simulink model "Local_trajectory_export"  (R2021a)
settings: configuration reference "AION_IDS_Speedgoat" (kept outside this file)
undefined symbols (not defined in the file): LATERAL_DISTANCE_THRESHOLD, MAX_GLOBAL_TRAJECTORY_WAY_POINT_NUMBER, MAX_LOCAL_TRAJECTORY_WAY_POINT_NUMBER, MAX_TRAJECTORY_LENGTH, START_END_DISTANCE_THRESHOLD
libraries: simulink x1
(part 1 of 2)
Description:
  | 局部轨迹导出模型
settings Model: DataDictionary=Local_Trajectory_Export.sldd  Creator=xinrui  LastModifiedBy=Administrator
settings ConfigSetRef: SourceName=AION_IDS_Speedgoat

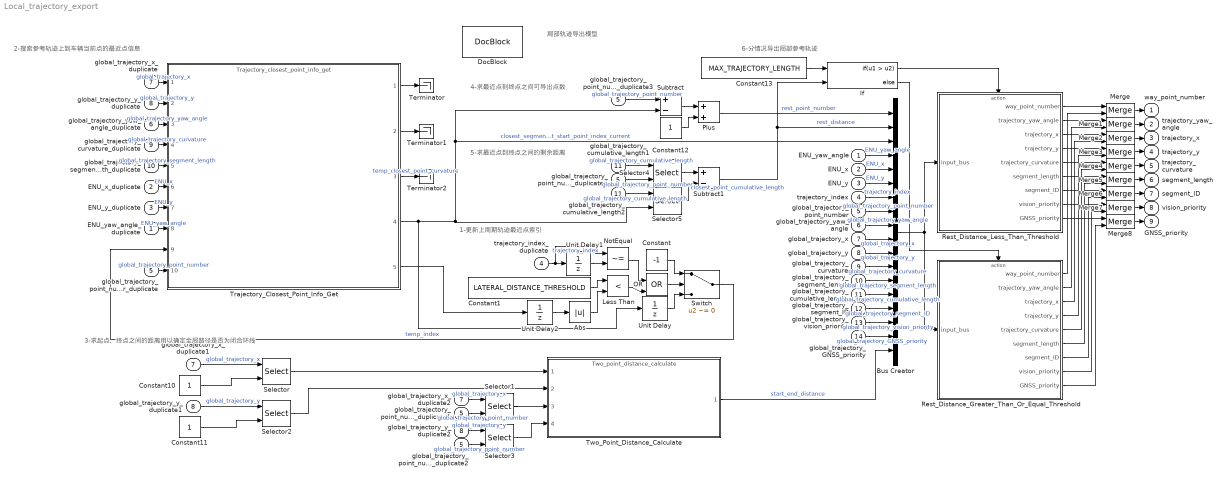
== system Local_trajectory_export ==
  note: 6-分情况导出局部参考轨迹
  note: 5-求最近点到终点之间的剩余距离
  note: 4-求最近点到终点之间可导出点数
  note: 1-更新上周期轨迹最近点索引
  note: 3-求起点、终点之间的距离用以确定全局路径是否为闭合环线
  note: 2-搜索参考轨迹上到车辆当前点的最近点信息
  note: 局部轨迹导出模型
  ENU_yaw_angle : Inport  Description=东北天坐标系下当前点横摆角，实数，deg。  OutDataTypeStr=double  PortDimensions=1
  ENU_x : Inport  Description=东北天坐标系下当前点x坐标，实数，m。  Port=2  OutDataTypeStr=double  PortDimensions=1
  ENU_y : Inport  Description=东北天坐标系下当前点y坐标，实数，m。  Port=3  OutDataTypeStr=double  PortDimensions=1
  trajectory_index : Inport  Description=选择的参考轨迹索引，正整数，无量纲。  Port=4  OutDataTypeStr=int8  PortDimensions=1
  global_trajectory_point_number : Inport  Description=选择的全局参考轨迹路点数量，正整数，无量纲。  Port=5  OutDataTypeStr=int32  PortDimensions=1
  global_trajectory_yaw_angle : Inport  Description=选择的全局参考轨迹横摆角数组，有效数据量为global_trajectory_point_number，实数，deg。  Port=6  OutDataTypeStr=double  PortDimensions=MAX_GLOBAL_TRAJECTORY_WAY_POINT_NUMBER  Interpolate=off
  global_trajectory_x : Inport  Description=选择的全局参考轨迹x坐标数组，有效数据量为global_trajectory_point_number，实数，m。  Port=7  OutDataTypeStr=double  PortDimensions=MAX_GLOBAL_TRAJECTORY_WAY_POINT_NUMBER  Interpolate=off
  global_trajectory_y : Inport  Description=选择的全局参考轨迹y坐标数组，有效数据量为global_trajectory_point_number，实数，m。  Port=8  OutDataTypeStr=double  PortDimensions=MAX_GLOBAL_TRAJECTORY_WAY_POINT_NUMBER  Interpolate=off
  global_trajectory_curvature : Inport  Description=选择的全局参考轨迹曲率数组，有效数据量为global_trajectory_point_number，实数，1/m。  Port=9  OutDataTypeStr=double  PortDimensions=MAX_GLOBAL_TRAJECTORY_WAY_POINT_NUMBER  Interpolate=off
  global_trajectory_segment_length : Inport  Description=选择的全局参考轨迹路点到前一个点的线段长度数组，有效数据量为global_trajectory_point_number，正实数，m。  Port=10  OutDataTypeStr=double  PortDimensions=MAX_GLOBAL_TRAJECTORY_WAY_POINT_NUMBER  Interpolate=off
  global_trajectory_cumulative_length : Inport  Description=选择的全局参考轨迹路点到起点的累计长度数组，有效数据量为global_trajectory_point_number，正实数，m。  Port=11  OutDataTypeStr=double  PortDimensions=MAX_GLOBAL_TRAJECTORY_WAY_POINT_NUMBER  Interpolate=off
  global_trajectory_segment_ID : Inport  Description=选择的全局参考轨迹区间代号数组，有效数据量为global_trajectory_point_number，正整数，无量纲。  Port=12  OutDataTypeStr=int8  PortDimensions=MAX_GLOBAL_TRAJECTORY_WAY_POINT_NUMBER  Interpolate=off
  global_trajectory_vision_priority : Inport  Description=选择的全局参考轨迹视觉循迹优先级数组，有效数据量为global_trajectory_point_number，自然数，无量纲。  Port=13  OutDataTypeStr=int8  PortDimensions=MAX_GLOBAL_TRAJECTORY_WAY_POINT_NUMBER  Interpolate=off
  global_trajectory_GNSS_priority : Inport  Description=选择的全局参考轨迹GNSS循迹优先级数组，有效数据量为global_trajectory_point_number，自然数，无量纲。  Port=14  OutDataTypeStr=int8  PortDimensions=MAX_GLOBAL_TRAJECTORY_WAY_POINT_NUMBER  Interpolate=off
  Abs : Abs
  Bus Creator : BusCreator  Inputs=18
  Constant : Constant  Value=-1  OutDataTypeStr=int32  SampleTime=-1
  Constant1 : Constant  Value=LATERAL_DISTANCE_THRESHOLD  OutDataTypeStr=double  SampleTime=-1
  Constant10 : Constant  OutDataTypeStr=int32  SampleTime=-1
  Constant11 : Constant  OutDataTypeStr=int32  SampleTime=-1
  Constant12 : Constant  OutDataTypeStr=int32  SampleTime=-1
  Constant13 : Constant  Value=MAX_TRAJECTORY_LENGTH  OutDataTypeStr=double  SampleTime=-1
  DocBlock : simulink/Model-Wide Utilities/DocBlock  DocumentType=HTML  mask(DocBlock){}
      mask Display:
      | plot([.8 0 0 1 1 .8 .8 1],[1 1 0 0 .8 1 .8 .8]);
      | text(.5,.6,'CHANGELOG','horizontalalignment','center');
      | text(.95,.05,get_param(gcb,'DocumentType'),'verticalalignment','bottom','horizontalalignment','right');
  ENU_x_duplicate : InportShadow  Description=东北天坐标系下当前点x坐标，实数，m。  Port=2  OutDataTypeStr=double  PortDimensions=1
  ENU_y_duplicate : InportShadow  Description=东北天坐标系下当前点y坐标，实数，m。  Port=3  OutDataTypeStr=double  PortDimensions=1
  ENU_yaw_angle_duplicate : InportShadow  Description=东北天坐标系下当前点横摆角，实数，deg。  OutDataTypeStr=double  PortDimensions=1
  If : If  Description=当最近点到终点之间累计距离不足最大轨迹长度的时候，判断起点、终点之间的距离。  NumInputs=2  IfExpression=u1 > u2
  Less Than : RelationalOperator  Operator=<  OutDataTypeStr=boolean  RndMeth=Simplest
  Merge{,1..8} (9 alike) : Merge
  NotEqual : RelationalOperator  Operator=~=  OutDataTypeStr=boolean  RndMeth=Simplest
  OR : Logic  Operator=OR  IconShape=distinctive  AllPortsSameDT=off  OutDataTypeStr=boolean
  Plus : Sum  Description=求最近点到终点之间可导出点数。
  Rest_Distance_Greater_Than_Or_Equal_Threshold : Subsystem  Description=当最近点到终点之间的累计距离大于最大轨迹长度的时候，按最大轨迹长度导出轨迹。  TreatAsAtomicUnit=on
  Rest_Distance_Less_Than_Threshold : Subsystem  Description=当最近点到终点之间累计距离不足最大轨迹长度的时候，判断起点、终点之间的距离。  TreatAsAtomicUnit=on
  Selector : Selector  Description=获取参考轨迹起点x坐标。  IndexOptions=Index vector (port)  Indices=[1 3]  OutputSizes=1
  Selector1 : Selector  Description=获取参考轨迹终点x坐标。  IndexOptions=Index vector (port)  Indices=[1 3]  OutputSizes=1
  Selector2 : Selector  Description=获取参考轨迹起点y坐标。  IndexOptions=Index vector (port)  Indices=[1 3]  OutputSizes=1
  Selector3 : Selector  Description=获取参考轨迹终点y坐标。  IndexOptions=Index vector (port)  Indices=[1 3]  OutputSizes=1
  Selector4 : Selector  Description=获取参考轨迹终点处的累计长度。  IndexOptions=Index vector (port)  Indices=[1 3]  OutputSizes=1
  Selector5 : Selector  Description=获取参考轨迹最近线段起始点处的累计长度。  IndexOptions=Index vector (port)  Indices=[1 3]  OutputSizes=1
  Subtract : Sum  Inputs=+-
  Subtract1 : Sum  Description=求最近点到终点之间的剩余距离。  Inputs=+-
  Switch : Switch  Description=|  Criteria=u2 ~= 0
      | 当以下任意条件满足时，采用全局搜索最近点，输入索引设置为-1，否则采用上周期的最近线段起始点索引作为本周期输入索引，使用局部搜索最近点信息。
      | （1）选定参考轨迹索引发生改变。
      | （2）近处横向偏差的绝对值大于阈值。
  Terminator : Terminator
  Terminator1 : Terminator
  Terminator2 : Terminator
  Trajectory_Closest_Point_Info_Get : ModelReference  Description=获取所选参考轨迹上的最近点信息。  ModelNameDialog=Trajectory_closest_point_info_get  SimulationMode=Normal  ModelReferenceVersion=4.338
  Two_Point_Distance_Calculate : ModelReference  Description=计算所选参考轨迹的起点和终点之间的距离，以判断参考轨迹是否为闭合环线。  ModelNameDialog=Two_point_distance_calculate  SimulationMode=Normal  ModelReferenceVersion=4.61
  Unit Delay : UnitDelay  InitialCondition=-1  SampleTime=-1  StateName=closest_segment_start_point_index_previous  HasFrameUpgradeWarning=on  StateMustResolveToSignalObject=on
  Unit Delay1 : UnitDelay  InitialCondition=-1  SampleTime=-1  StateName=trajectory_index_previous  HasFrameUpgradeWarning=on  StateMustResolveToSignalObject=on
  Unit Delay2 : UnitDelay  SampleTime=-1  StateName=near_lateral_offset_previous  HasFrameUpgradeWarning=on  StateMustResolveToSignalObject=on
  global_trajectory_cumulative_length1 : InportShadow  Description=选择的全局参考轨迹路点到起点的累计长度数组，有效数据量为global_trajectory_point_number，正实数，m。  Port=11  OutDataTypeStr=double  PortDimensions=MAX_GLOBAL_TRAJECTORY_WAY_POINT_NUMBER  Interpolate=off
  global_trajectory_cumulative_length2 : InportShadow  Description=选择的全局参考轨迹路点到起点的累计长度数组，有效数据量为global_trajectory_point_number，正实数，m。  Port=11  OutDataTypeStr=double  PortDimensions=MAX_GLOBAL_TRAJECTORY_WAY_POINT_NUMBER  Interpolate=off
  global_trajectory_curvature_duplicate : InportShadow  Description=选择的全局参考轨迹曲率数组，有效数据量为global_trajectory_point_number，实数，1/m。  Port=9  OutDataTypeStr=double  PortDimensions=MAX_GLOBAL_TRAJECTORY_WAY_POINT_NUMBER  Interpolate=off
  global_trajectory_point_number_duplicate{,1..4} (5 alike) : InportShadow  Description=选择的全局参考轨迹路点数量，正整数，无量纲。  Port=5  OutDataTypeStr=int32  PortDimensions=1
  global_trajectory_segment_length_duplicate : InportShadow  Description=选择的全局参考轨迹路点到前一个点的线段长度数组，有效数据量为global_trajectory_point_number，正实数，m。  Port=10  OutDataTypeStr=double  PortDimensions=MAX_GLOBAL_TRAJECTORY_WAY_POINT_NUMBER  Interpolate=off
  global_trajectory_x_duplicate : InportShadow  Description=选择的全局参考轨迹x坐标数组，有效数据量为global_trajectory_point_number，实数，m。  Port=7  OutDataTypeStr=double  PortDimensions=MAX_GLOBAL_TRAJECTORY_WAY_POINT_NUMBER  Interpolate=off
  global_trajectory_x_duplicate1 : InportShadow  Description=选择的全局参考轨迹x坐标数组，有效数据量为global_trajectory_point_number，实数，m。  Port=7  OutDataTypeStr=double  PortDimensions=MAX_GLOBAL_TRAJECTORY_WAY_POINT_NUMBER  Interpolate=off
  global_trajectory_x_duplicate2 : InportShadow  Description=选择的全局参考轨迹x坐标数组，有效数据量为global_trajectory_point_number，实数，m。  Port=7  OutDataTypeStr=double  PortDimensions=MAX_GLOBAL_TRAJECTORY_WAY_POINT_NUMBER  Interpolate=off
  global_trajectory_y_duplicate : InportShadow  Description=选择的全局参考轨迹y坐标数组，有效数据量为global_trajectory_point_number，实数，m。  Port=8  OutDataTypeStr=double  PortDimensions=MAX_GLOBAL_TRAJECTORY_WAY_POINT_NUMBER  Interpolate=off
  global_trajectory_y_duplicate1 : InportShadow  Description=选择的全局参考轨迹y坐标数组，有效数据量为global_trajectory_point_number，实数，m。  Port=8  OutDataTypeStr=double  PortDimensions=MAX_GLOBAL_TRAJECTORY_WAY_POINT_NUMBER  Interpolate=off
  global_trajectory_y_duplicate2 : InportShadow  Description=选择的全局参考轨迹y坐标数组，有效数据量为global_trajectory_point_number，实数，m。  Port=8  OutDataTypeStr=double  PortDimensions=MAX_GLOBAL_TRAJECTORY_WAY_POINT_NUMBER  Interpolate=off
  global_trajectory_yaw_angle_duplicate : InportShadow  Description=选择的全局参考轨迹横摆角数组，有效数据量为global_trajectory_point_number，实数，deg。  Port=6  OutDataTypeStr=double  PortDimensions=MAX_GLOBAL_TRAJECTORY_WAY_POINT_NUMBER  Interpolate=off
  trajectory_index_duplicate : InportShadow  Description=选择的参考轨迹索引，正整数，无量纲。  Port=4  OutDataTypeStr=int8  PortDimensions=1
  way_point_number : Outport  Description=导出的局部轨迹有效路点个数，自然数，无量纲。  OutDataTypeStr=int32  PortDimensions=1
  trajectory_yaw_angle : Outport  Description=导出的局部轨迹横摆角数组，有效数据数量为way_point_number，其余补零，实数，deg。  Port=2  OutDataTypeStr=double  PortDimensions=MAX_LOCAL_TRAJECTORY_WAY_POINT_NUMBER
  trajectory_x : Outport  Description=导出的局部轨迹x坐标数组，有效数据数量为way_point_number，其余补零，实数，m。  Port=3  OutDataTypeStr=double  PortDimensions=MAX_LOCAL_TRAJECTORY_WAY_POINT_NUMBER
  trajectory_y : Outport  Description=导出的局部轨迹y坐标数组，有效数据数量为way_point_number，其余补零，实数，m。  Port=4  OutDataTypeStr=double  PortDimensions=MAX_LOCAL_TRAJECTORY_WAY_POINT_NUMBER
  trajectory_curvature : Outport  Description=导出的局部轨迹曲率数组，有效数据数量为way_point_number，其余补零，实数，1/m。  Port=5  OutDataTypeStr=double  PortDimensions=MAX_LOCAL_TRAJECTORY_WAY_POINT_NUMBER
  segment_length : Outport  Description=导出的局部轨迹路点到前一个点的线段长度数组，有效数据数量为way_point_number，其余补零，正实数，m。  Port=6  OutDataTypeStr=double  PortDimensions=MAX_LOCAL_TRAJECTORY_WAY_POINT_NUMBER
  segment_ID : Outport  Description=导出的局部轨迹区间代号数组，有效数据数量为way_point_number，其余补零，正整数，无量纲。  Port=7  OutDataTypeStr=int8  PortDimensions=MAX_LOCAL_TRAJECTORY_WAY_POINT_NUMBER
  vision_priority : Outport  Description=导出的局部轨迹视觉循迹优先级数组，有效数据数量为way_point_number，其余补零，自然数，无量纲。  Port=8  OutDataTypeStr=int8  PortDimensions=MAX_LOCAL_TRAJECTORY_WAY_POINT_NUMBER
  GNSS_priority : Outport  Description=导出的局部轨迹GNSS循迹优先级数组，有效数据数量为way_point_number，其余补零，自然数，无量纲。  Port=9  OutDataTypeStr=int8  PortDimensions=MAX_LOCAL_TRAJECTORY_WAY_POINT_NUMBER
  wires:
  trajectory_index_duplicate/1 -> NotEqual/1, Unit Delay1/1  "trajectory_index"
  Switch/1 -> Trajectory_Closest_Point_Info_Get/9  "temp_index"
  Constant/1 -> Switch/1
  Trajectory_Closest_Point_Info_Get/4 -> Unit Delay/1, Subtract/2, Bus Creator/3, Selector5/2  "closest_segment_start_point_index_current"
  Unit Delay/1 -> Switch/3
  global_trajectory_x_duplicate/1 -> Trajectory_Closest_Point_Info_Get/1  "global_trajectory_x"
  global_trajectory_y_duplicate/1 -> Trajectory_Closest_Point_Info_Get/2  "global_trajectory_y"
  global_trajectory_yaw_angle_duplicate/1 -> Trajectory_Closest_Point_Info_Get/3  "global_trajectory_yaw_angle"
  global_trajectory_curvature_duplicate/1 -> Trajectory_Closest_Point_Info_Get/4  "global_trajectory_curvature"
  global_trajectory_segment_length_duplicate/1 -> Trajectory_Closest_Point_Info_Get/5  "global_trajectory_segment_length"
  ENU_x_duplicate/1 -> Trajectory_Closest_Point_Info_Get/6  "ENU_x"
  ENU_y_duplicate/1 -> Trajectory_Closest_Point_Info_Get/7  "ENU_y"
  ENU_yaw_angle_duplicate/1 -> Trajectory_Closest_Point_Info_Get/8  "ENU_yaw_angle"
  global_trajectory_point_number_duplicate/1 -> Trajectory_Closest_Point_Info_Get/10  "global_trajectory_point_number"
  Unit Delay1/1 -> NotEqual/2
  global_trajectory_x_duplicate1/1 -> Selector/1  "global_trajectory_x"
  Constant10/1 -> Selector/2
  Selector/1 -> Two_Point_Distance_Calculate/1
  global_trajectory_point_number_duplicate1/1 -> Selector1/2  "global_trajectory_point_number"
  global_trajectory_x_duplicate2/1 -> Selector1/1  "global_trajectory_x"
  Selector1/1 -> Two_Point_Distance_Calculate/3
  Constant11/1 -> Selector2/2
  global_trajectory_y_duplicate1/1 -> Selector2/1  "global_trajectory_y"
  Selector2/1 -> Two_Point_Distance_Calculate/2
  global_trajectory_y_duplicate2/1 -> Selector3/1  "global_trajectory_y"
  global_trajectory_point_number_duplicate2/1 -> Selector3/2  "global_trajectory_point_number"
  Selector3/1 -> Two_Point_Distance_Calculate/4
  global_trajectory_point_number_duplicate3/1 -> Subtract/1  "global_trajectory_point_number"
  Subtract/1 -> Plus/1
  Constant12/1 -> Plus/2
  global_trajectory_cumulative_length1/1 -> Selector4/1  "global_trajectory_cumulative_length"
  global_trajectory_point_number_duplicate4/1 -> Selector4/2  "global_trajectory_point_number"
  global_trajectory_cumulative_length2/1 -> Selector5/1  "global_trajectory_cumulative_length"
  Selector4/1 -> Subtract1/1
  Selector5/1 -> Subtract1/2  "closest_point_cumulative_length"
  Subtract1/1 -> Bus Creator/2, If/2  "rest_distance"
  Plus/1 -> Bus Creator/1  "rest_point_number"
  Two_Point_Distance_Calculate/1 -> Bus Creator/18  "start_end_distance"
  ENU_yaw_angle/1 -> Bus Creator/4  "ENU_yaw_angle"
  ENU_x/1 -> Bus Creator/5  "ENU_x"
  ENU_y/1 -> Bus Creator/6  "ENU_y"
  trajectory_index/1 -> Bus Creator/7  "trajectory_index"
  global_trajectory_point_number/1 -> Bus Creator/8  "global_trajectory_point_number"
  global_trajectory_yaw_angle/1 -> Bus Creator/9  "global_trajectory_yaw_angle"
  global_trajectory_x/1 -> Bus Creator/10  "global_trajectory_x"
  global_trajectory_y/1 -> Bus Creator/11  "global_trajectory_y"
  global_trajectory_curvature/1 -> Bus Creator/12  "global_trajectory_curvature"
  global_trajectory_segment_length/1 -> Bus Creator/13  "global_trajectory_segment_length"
  global_trajectory_cumulative_length/1 -> Bus Creator/14  "global_trajectory_cumulative_length"
  global_trajectory_segment_ID/1 -> Bus Creator/15  "global_trajectory_segment_ID"
  global_trajectory_vision_priority/1 -> Bus Creator/16  "global_trajectory_vision_priority"
  global_trajectory_GNSS_priority/1 -> Bus Creator/17  "global_trajectory_GNSS_priority"
  Constant13/1 -> If/1
  If/1 -> Rest_Distance_Less_Than_Threshold/Action
  Bus Creator/1 -> Rest_Distance_Greater_Than_Or_Equal_Threshold/1(input_bus), Rest_Distance_Less_Than_Threshold/1(input_bus)
  If/2 -> Rest_Distance_Greater_Than_Or_Equal_Threshold/Action
  Merge/1 -> way_point_number/1
  Rest_Distance_Less_Than_Threshold/1(way_point_number) -> Merge/1
  Rest_Distance_Greater_Than_Or_Equal_Threshold/1(way_point_number) -> Merge/2
  Merge1/1 -> trajectory_yaw_angle/1
  Rest_Distance_Less_Than_Threshold/2(trajectory_yaw_angle) -> Merge1/1
  Rest_Distance_Greater_Than_Or_Equal_Threshold/2(trajectory_yaw_angle) -> Merge1/2
  Merge2/1 -> trajectory_x/1
  Rest_Distance_Less_Than_Threshold/3(trajectory_x) -> Merge2/1
  Rest_Distance_Greater_Than_Or_Equal_Threshold/3(trajectory_x) -> Merge2/2
  Merge3/1 -> trajectory_y/1
  Rest_Distance_Less_Than_Threshold/4(trajectory_y) -> Merge3/1
  Rest_Distance_Greater_Than_Or_Equal_Threshold/4(trajectory_y) -> Merge3/2
  Rest_Distance_Less_Than_Threshold/5(trajectory_curvature) -> Merge4/1
  Rest_Distance_Greater_Than_Or_Equal_Threshold/5(trajectory_curvature) -> Merge4/2
  Merge4/1 -> trajectory_curvature/1
  Merge5/1 -> segment_length/1
  Rest_Distance_Less_Than_Threshold/6(segment_length) -> Merge5/1
  Rest_Distance_Greater_Than_Or_Equal_Threshold/6(segment_length) -> Merge5/2
  Merge6/1 -> segment_ID/1
  Rest_Distance_Less_Than_Threshold/7(segment_ID) -> Merge6/1
  Rest_Distance_Greater_Than_Or_Equal_Threshold/7(segment_ID) -> Merge6/2
  Rest_Distance_Less_Than_Threshold/8(vision_priority) -> Merge7/1
  Rest_Distance_Greater_Than_Or_Equal_Threshold/8(vision_priority) -> Merge7/2
  Merge7/1 -> vision_priority/1
  Merge8/1 -> GNSS_priority/1
  Rest_Distance_Less_Than_Threshold/9(GNSS_priority) -> Merge8/1
  Rest_Distance_Greater_Than_Or_Equal_Threshold/9(GNSS_priority) -> Merge8/2
  OR/1 -> Switch/2
  NotEqual/1 -> OR/1
  Constant1/1 -> Less Than/1
  Less Than/1 -> OR/2
  Trajectory_Closest_Point_Info_Get/5 -> Unit Delay2/1
  Trajectory_Closest_Point_Info_Get/1 -> Terminator/1
  Trajectory_Closest_Point_Info_Get/2 -> Terminator1/1
  Trajectory_Closest_Point_Info_Get/3 -> Terminator2/1  "temp_closest_point_curvature"
  Abs/1 -> Less Than/2
  Unit Delay2/1 -> Abs/1

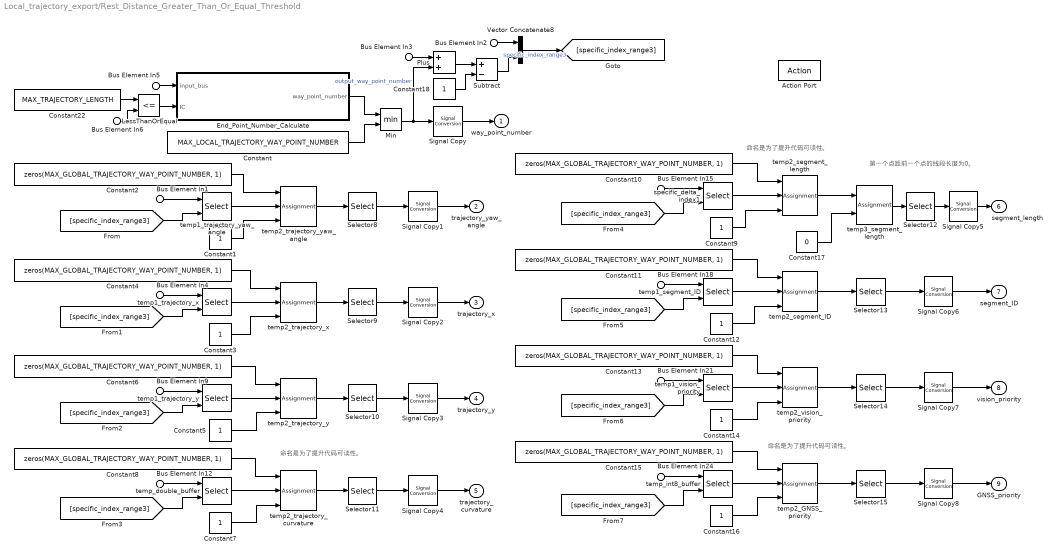
== system Local_trajectory_export/Rest_Distance_Greater_Than_Or_Equal_Threshold ==
  note: 命名是为了提升代码可读性。
  note: 第一个点距前一个点的线段长度为0。
  note: 命名是为了提升代码可读性。
  note: 命名是为了提升代码可读性。
  Bus Element In5 : Inport  PortName=input_bus
  Bus Element In6 : Inport  PortName=input_bus  Element=rest_distance
  Bus Element In1 : Inport  PortName=input_bus  Element=global_trajectory_yaw_angle
  Bus Element In2 : Inport  PortName=input_bus  Element=closest_segment_start_point_index_current
  Bus Element In3 : Inport  PortName=input_bus  Element=closest_segment_start_point_index_current
  Bus Element In4 : Inport  PortName=input_bus  Element=global_trajectory_x
  Bus Element In9 : Inport  PortName=input_bus  Element=global_trajectory_y
  Bus Element In12 : Inport  PortName=input_bus  Element=global_trajectory_curvature
  Bus Element In15 : Inport  PortName=input_bus  Element=global_trajectory_segment_length
  Bus Element In18 : Inport  PortName=input_bus  Element=global_trajectory_segment_ID
  Bus Element In21 : Inport  PortName=input_bus  Element=global_trajectory_vision_priority
  Bus Element In24 : Inport  PortName=input_bus  Element=global_trajectory_GNSS_priority
  Action Port : ActionPort  PropagateVarSize=During execution  ActionPortLabel=else
  Constant : Constant  Value=MAX_LOCAL_TRAJECTORY_WAY_POINT_NUMBER  VectorParams1D=off  OutDataTypeStr=int32  SampleTime=-1
  Constant{1,3,5,7,9,12,14,16,18} (9 alike) : Constant  OutDataTypeStr=int32  SampleTime=-1
  Constant{2,4,6,8,10} (5 alike) : Constant  Value=zeros(MAX_GLOBAL_TRAJECTORY_WAY_POINT_NUMBER, 1)  OutDataTypeStr=double  SampleTime=-1
  Constant11 : Constant  Value=zeros(MAX_GLOBAL_TRAJECTORY_WAY_POINT_NUMBER, 1)  OutDataTypeStr=int8  SampleTime=-1
  Constant13 : Constant  Value=zeros(MAX_GLOBAL_TRAJECTORY_WAY_POINT_NUMBER, 1)  OutDataTypeStr=int8  SampleTime=-1
  Constant15 : Constant  Value=zeros(MAX_GLOBAL_TRAJECTORY_WAY_POINT_NUMBER, 1)  OutDataTypeStr=int8  SampleTime=-1
  Constant17 : Constant  Value=0  OutDataTypeStr=double  SampleTime=-1
  Constant22 : Constant  Value=MAX_TRAJECTORY_LENGTH  OutDataTypeStr=double  SampleTime=-1
  End_Point_Number_Calculate : Subsystem  Description=遍历搜索满足导出轨迹累计弧长条件的从最近点往后的点数。  TreatAsAtomicUnit=on
  LessThanOrEqual : RelationalOperator  Operator=<=  OutDataTypeStr=boolean  RndMeth=Simplest
  Min : MinMax  Inputs=2  OutDataTypeStr=int32
  Plus : Sum
  Selector{8..15} (8 alike) : Selector  IndexOptions=Starting index (dialog)  Indices=1  OutputSizes=MAX_LOCAL_TRAJECTORY_WAY_POINT_NUMBER
  Signal Copy{,1..8} (9 alike) : SignalConversion  OverrideOpt=off
  Subtract : Sum  Inputs=+-
  Vector Concatenate8 : Concatenate
  specific_delta_index1 : Selector  IndexOptions=Starting and ending indices (port)  Indices=[1 3]  OutputSizes=MAX_LOCAL_TRAJECTORY_WAY_POINT_NUMBER
  temp1_segment_ID : Selector  IndexOptions=Starting and ending indices (port)  Indices=[1 3]  OutputSizes=MAX_LOCAL_TRAJECTORY_WAY_POINT_NUMBER
  temp1_trajectory_x : Selector  IndexOptions=Starting and ending indices (port)  Indices=[1 3]  OutputSizes=MAX_LOCAL_TRAJECTORY_WAY_POINT_NUMBER
  temp1_trajectory_y : Selector  IndexOptions=Starting and ending indices (port)  Indices=[1 3]  OutputSizes=MAX_LOCAL_TRAJECTORY_WAY_POINT_NUMBER
  temp1_trajectory_yaw_angle : Selector  IndexOptions=Starting and ending indices (port)  Indices=[1 3]  OutputSizes=MAX_LOCAL_TRAJECTORY_WAY_POINT_NUMBER
  temp1_vision_priority : Selector  IndexOptions=Starting and ending indices (port)  Indices=[1 3]  OutputSizes=MAX_LOCAL_TRAJECTORY_WAY_POINT_NUMBER
  temp2_GNSS_priority : Assignment  DiagnosticForDimensions=Warning  IndexOptions=Starting index (port)  Indices=1  OutputSizes=MAX_LOCAL_TRAJECTORY_WAY_POINT_NUMBER
  temp2_segment_ID : Assignment  DiagnosticForDimensions=Warning  IndexOptions=Starting index (port)  Indices=1  OutputSizes=MAX_LOCAL_TRAJECTORY_WAY_POINT_NUMBER
  temp2_segment_length : Assignment  DiagnosticForDimensions=Warning  IndexOptions=Starting index (port)  Indices=1  OutputSizes=MAX_LOCAL_TRAJECTORY_WAY_POINT_NUMBER
  temp2_trajectory_curvature : Assignment  DiagnosticForDimensions=Warning  IndexOptions=Starting index (port)  Indices=1  OutputSizes=MAX_LOCAL_TRAJECTORY_WAY_POINT_NUMBER
  temp2_trajectory_x : Assignment  DiagnosticForDimensions=Warning  IndexOptions=Starting index (port)  Indices=1  OutputSizes=MAX_LOCAL_TRAJECTORY_WAY_POINT_NUMBER
  temp2_trajectory_y : Assignment  DiagnosticForDimensions=Warning  IndexOptions=Starting index (port)  Indices=1  OutputSizes=MAX_LOCAL_TRAJECTORY_WAY_POINT_NUMBER
  temp2_trajectory_yaw_angle : Assignment  DiagnosticForDimensions=Warning  IndexOptions=Starting index (port)  Indices=1  OutputSizes=MAX_LOCAL_TRAJECTORY_WAY_POINT_NUMBER
  temp2_vision_priority : Assignment  DiagnosticForDimensions=Warning  IndexOptions=Starting index (port)  Indices=1  OutputSizes=MAX_LOCAL_TRAJECTORY_WAY_POINT_NUMBER
  temp3_segment_length : Assignment  Description=第一个点距前一个点的线段长度为0。  OutputInitialize=Specify size for each dimension in table  DiagnosticForDimensions=Warning  IndexOptions=Index vector (dialog)  Indices=1  OutputSizes=MAX_LOCAL_TRAJECTORY_WAY_POINT_NUMBER
  temp_double_buffer : Selector  IndexOptions=Starting and ending indices (port)  Indices=[1 3]  OutputSizes=MAX_LOCAL_TRAJECTORY_WAY_POINT_NUMBER
  temp_int8_buffer : Selector  IndexOptions=Starting and ending indices (port)  Indices=[1 3]  OutputSizes=MAX_LOCAL_TRAJECTORY_WAY_POINT_NUMBER
  way_point_number : Outport  Description=导出的局部轨迹有效路点个数，自然数，无量纲。  OutDataTypeStr=int32  PortDimensions=1
  trajectory_yaw_angle : Outport  Description=导出的局部轨迹横摆角数组，有效数据数量为way_point_number，其余补零，实数，deg。  Port=2  OutDataTypeStr=double  PortDimensions=MAX_LOCAL_TRAJECTORY_WAY_POINT_NUMBER
  trajectory_x : Outport  Description=导出的局部轨迹x坐标数组，有效数据数量为way_point_number，其余补零，实数，m。  Port=3  OutDataTypeStr=double  PortDimensions=MAX_LOCAL_TRAJECTORY_WAY_POINT_NUMBER
  trajectory_y : Outport  Description=导出的局部轨迹y坐标数组，有效数据数量为way_point_number，其余补零，实数，m。  Port=4  OutDataTypeStr=double  PortDimensions=MAX_LOCAL_TRAJECTORY_WAY_POINT_NUMBER
  trajectory_curvature : Outport  Description=导出的局部轨迹曲率数组，有效数据数量为way_point_number，其余补零，实数，1/m。  Port=5  OutDataTypeStr=double  PortDimensions=MAX_LOCAL_TRAJECTORY_WAY_POINT_NUMBER
  segment_length : Outport  Description=导出的局部轨迹路点到前一个点的线段长度数组，有效数据数量为way_point_number，其余补零，正实数，m。  Port=6  OutDataTypeStr=double  PortDimensions=MAX_LOCAL_TRAJECTORY_WAY_POINT_NUMBER
  segment_ID : Outport  Description=导出的局部轨迹区间代号数组，有效数据数量为way_point_number，其余补零，正整数，无量纲。  Port=7  OutDataTypeStr=int8  PortDimensions=MAX_LOCAL_TRAJECTORY_WAY_POINT_NUMBER
  vision_priority : Outport  Description=导出的局部轨迹视觉循迹优先级数组，有效数据数量为way_point_number，其余补零，自然数，无量纲。  Port=8  OutDataTypeStr=int8  PortDimensions=MAX_LOCAL_TRAJECTORY_WAY_POINT_NUMBER
  GNSS_priority : Outport  Description=导出的局部轨迹GNSS循迹优先级数组，有效数据数量为way_point_number，其余补零，自然数，无量纲。  Port=9  OutDataTypeStr=int8  PortDimensions=MAX_LOCAL_TRAJECTORY_WAY_POINT_NUMBER
  wires:
  Min/1 -> Signal Copy/1, Plus/2  "output_way_point_number"
  Constant/1 -> Min/2
  Bus Element In5/1 -> End_Point_Number_Calculate/1(input_bus)
  End_Point_Number_Calculate/1(way_point_number) -> Min/1
  Constant22/1 -> LessThanOrEqual/1
  Bus Element In6/1 -> LessThanOrEqual/2
  LessThanOrEqual/1 -> End_Point_Number_Calculate/2(IC)
  Signal Copy/1 -> way_point_number/1
  Signal Copy5/1 -> segment_length/1
  Signal Copy6/1 -> segment_ID/1
  temp2_trajectory_yaw_angle/1 -> Selector8/1
  Constant7/1 -> temp2_trajectory_curvature/3
  Signal Copy4/1 -> trajectory_curvature/1
  Bus Element In1/1 -> temp1_trajectory_yaw_angle/1
  temp1_trajectory_x/1 -> temp2_trajectory_x/2
  temp1_segment_ID/1 -> temp2_segment_ID/2
  temp2_vision_priority/1 -> Selector14/1
  temp2_trajectory_curvature/1 -> Selector11/1
  [specific_index_range3] -> temp1_vision_priority/2
  Selector8/1 -> Signal Copy1/1
  Signal Copy3/1 -> trajectory_y/1
  Selector12/1 -> Signal Copy5/1
  specific_delta_index1/1 -> temp2_segment_length/2
  Vector Concatenate8/1 -> [specific_index_range3]  "specific_index_range3"
  temp3_segment_length/1 -> Selector12/1
  temp2_segment_ID/1 -> Selector13/1
  Constant17/1 -> temp3_segment_length/2
  Bus Element In3/1 -> Plus/1
  temp2_GNSS_priority/1 -> Selector15/1
  Signal Copy2/1 -> trajectory_x/1
  Constant2/1 -> temp2_trajectory_yaw_angle/1
  Plus/1 -> Subtract/1
  Constant18/1 -> Subtract/2
  temp_int8_buffer/1 -> temp2_GNSS_priority/2
  [specific_index_range3] -> specific_delta_index1/2
  [specific_index_range3] -> temp_int8_buffer/2
  Constant15/1 -> temp2_GNSS_priority/1
  Constant13/1 -> temp2_vision_priority/1
  Bus Element In2/1 -> Vector Concatenate8/1
  Bus Element In9/1 -> temp1_trajectory_y/1
  [specific_index_range3] -> temp1_trajectory_y/2
  Constant8/1 -> temp2_trajectory_curvature/1
  [specific_index_range3] -> temp_double_buffer/2
  Constant4/1 -> temp2_trajectory_x/1
  temp2_trajectory_x/1 -> Selector9/1
  Bus Element In21/1 -> temp1_vision_priority/1
  Bus Element In18/1 -> temp1_segment_ID/1
  Bus Element In4/1 -> temp1_trajectory_x/1
  Bus Element In15/1 -> specific_delta_index1/1
  temp2_trajectory_y/1 -> Selector10/1
  Signal Copy8/1 -> GNSS_priority/1
  Selector10/1 -> Signal Copy3/1
  [specific_index_range3] -> temp1_segment_ID/2
  Constant11/1 -> temp2_segment_ID/1
  Selector13/1 -> Signal Copy6/1
  [specific_index_range3] -> temp1_trajectory_yaw_angle/2
  Signal Copy1/1 -> trajectory_yaw_angle/1
  Bus Element In12/1 -> temp_double_buffer/1
  temp1_vision_priority/1 -> temp2_vision_priority/2
  Bus Element In24/1 -> temp_int8_buffer/1
  Selector15/1 -> Signal Copy8/1
  Constant12/1 -> temp2_segment_ID/3
  Constant1/1 -> temp2_trajectory_yaw_angle/3
  temp1_trajectory_yaw_angle/1 -> temp2_trajectory_yaw_angle/2
  Selector11/1 -> Signal Copy4/1
  Selector14/1 -> Signal Copy7/1
  Selector9/1 -> Signal Copy2/1
  Constant6/1 -> temp2_trajectory_y/1
  Subtract/1 -> Vector Concatenate8/2
  [specific_index_range3] -> temp1_trajectory_x/2
  Constant16/1 -> temp2_GNSS_priority/3
  Constant3/1 -> temp2_trajectory_x/3
  Constant9/1 -> temp2_segment_length/3
  temp_double_buffer/1 -> temp2_trajectory_curvature/2
  Constant14/1 -> temp2_vision_priority/3
  temp2_segment_length/1 -> temp3_segment_length/1
  temp1_trajectory_y/1 -> temp2_trajectory_y/2
  Constant10/1 -> temp2_segment_length/1
  Constant5/1 -> temp2_trajectory_y/3
  Signal Copy7/1 -> vision_priority/1

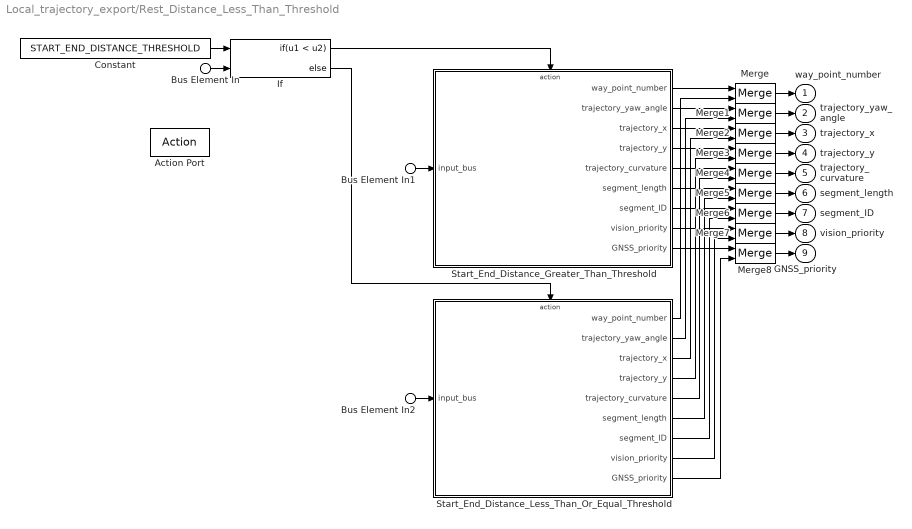
== system Local_trajectory_export/Rest_Distance_Less_Than_Threshold ==
  Bus Element In1 : Inport  PortName=input_bus
  Bus Element In2 : Inport  PortName=input_bus
  Bus Element In : Inport  PortName=input_bus  Element=start_end_distance
  Action Port : ActionPort  PropagateVarSize=During execution  ActionPortLabel=if(u1 > u2)
  Constant : Constant  Value=START_END_DISTANCE_THRESHOLD  OutDataTypeStr=double  SampleTime=-1
  If : If  Description=起点、终点之间的距离大于阈值，非闭合环线，直接从最近点导出到终点。  NumInputs=2  IfExpression=u1 < u2
  Merge{,1..8} (9 alike) : Merge
  Start_End_Distance_Greater_Than_Threshold : Subsystem  Description=起点、终点之间的距离大于阈值，非闭合环线，直接从最近点导出到终点。  TreatAsAtomicUnit=on
  Start_End_Distance_Less_Than_Or_Equal_Threshold : Subsystem  Description=起点、终点之间的距离小于等于阈值，闭合环线，从最近点导出到终点之后，接续从起点到剩余点的轨迹。  TreatAsAtomicUnit=on
  way_point_number : Outport  Description=导出的局部轨迹有效路点个数，自然数，无量纲。  OutDataTypeStr=int32  PortDimensions=1
  trajectory_yaw_angle : Outport  Description=导出的局部轨迹横摆角数组，有效数据数量为way_point_number，其余补零，实数，deg。  Port=2  OutDataTypeStr=double  PortDimensions=MAX_LOCAL_TRAJECTORY_WAY_POINT_NUMBER
  trajectory_x : Outport  Description=导出的局部轨迹x坐标数组，有效数据数量为way_point_number，其余补零，实数，m。  Port=3  OutDataTypeStr=double  PortDimensions=MAX_LOCAL_TRAJECTORY_WAY_POINT_NUMBER
  trajectory_y : Outport  Description=导出的局部轨迹y坐标数组，有效数据数量为way_point_number，其余补零，实数，m。  Port=4  OutDataTypeStr=double  PortDimensions=MAX_LOCAL_TRAJECTORY_WAY_POINT_NUMBER
  trajectory_curvature : Outport  Description=导出的局部轨迹曲率数组，有效数据数量为way_point_number，其余补零，实数，1/m。  Port=5  OutDataTypeStr=double  PortDimensions=MAX_LOCAL_TRAJECTORY_WAY_POINT_NUMBER
  segment_length : Outport  Description=导出的局部轨迹路点到前一个点的线段长度数组，有效数据数量为way_point_number，其余补零，正实数，m。  Port=6  OutDataTypeStr=double  PortDimensions=MAX_LOCAL_TRAJECTORY_WAY_POINT_NUMBER
  segment_ID : Outport  Description=导出的局部轨迹区间代号数组，有效数据数量为way_point_number，其余补零，正整数，无量纲。  Port=7  OutDataTypeStr=int8  PortDimensions=MAX_LOCAL_TRAJECTORY_WAY_POINT_NUMBER
  vision_priority : Outport  Description=导出的局部轨迹视觉循迹优先级数组，有效数据数量为way_point_number，其余补零，自然数，无量纲。  Port=8  OutDataTypeStr=int8  PortDimensions=MAX_LOCAL_TRAJECTORY_WAY_POINT_NUMBER
  GNSS_priority : Outport  Description=导出的局部轨迹GNSS循迹优先级数组，有效数据数量为way_point_number，其余补零，自然数，无量纲。  Port=9  OutDataTypeStr=int8  PortDimensions=MAX_LOCAL_TRAJECTORY_WAY_POINT_NUMBER
  wires:
  Bus Element In/1 -> If/2
  Constant/1 -> If/1
  If/1 -> Start_End_Distance_Greater_Than_Threshold/Action
  Bus Element In1/1 -> Start_End_Distance_Greater_Than_Threshold/1(input_bus)
  Bus Element In2/1 -> Start_End_Distance_Less_Than_Or_Equal_Threshold/1(input_bus)
  If/2 -> Start_End_Distance_Less_Than_Or_Equal_Threshold/Action
  Merge/1 -> way_point_number/1
  Start_End_Distance_Greater_Than_Threshold/1(way_point_number) -> Merge/1
  Start_End_Distance_Less_Than_Or_Equal_Threshold/1(way_point_number) -> Merge/2
  Merge1/1 -> trajectory_yaw_angle/1
  Start_End_Distance_Greater_Than_Threshold/2(trajectory_yaw_angle) -> Merge1/1
  Start_End_Distance_Less_Than_Or_Equal_Threshold/2(trajectory_yaw_angle) -> Merge1/2
  Merge2/1 -> trajectory_x/1
  Start_End_Distance_Greater_Than_Threshold/3(trajectory_x) -> Merge2/1
  Start_End_Distance_Less_Than_Or_Equal_Threshold/3(trajectory_x) -> Merge2/2
  Merge3/1 -> trajectory_y/1
  Start_End_Distance_Greater_Than_Threshold/4(trajectory_y) -> Merge3/1
  Start_End_Distance_Less_Than_Or_Equal_Threshold/4(trajectory_y) -> Merge3/2
  Merge4/1 -> trajectory_curvature/1
  Start_End_Distance_Greater_Than_Threshold/5(trajectory_curvature) -> Merge4/1
  Start_End_Distance_Less_Than_Or_Equal_Threshold/5(trajectory_curvature) -> Merge4/2
  Merge5/1 -> segment_length/1
  Start_End_Distance_Greater_Than_Threshold/6(segment_length) -> Merge5/1
  Start_End_Distance_Less_Than_Or_Equal_Threshold/6(segment_length) -> Merge5/2
  Merge6/1 -> segment_ID/1
  Start_End_Distance_Greater_Than_Threshold/7(segment_ID) -> Merge6/1
  Start_End_Distance_Less_Than_Or_Equal_Threshold/7(segment_ID) -> Merge6/2
  Merge7/1 -> vision_priority/1
  Start_End_Distance_Greater_Than_Threshold/8(vision_priority) -> Merge7/1
  Start_End_Distance_Less_Than_Or_Equal_Threshold/8(vision_priority) -> Merge7/2
  Merge8/1 -> GNSS_priority/1
  Start_End_Distance_Greater_Than_Threshold/9(GNSS_priority) -> Merge8/1
  Start_End_Distance_Less_Than_Or_Equal_Threshold/9(GNSS_priority) -> Merge8/2

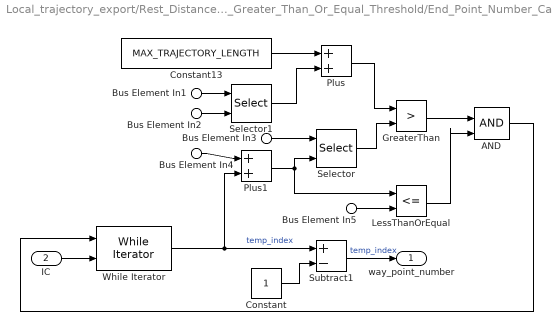
== system Local_trajectory_export/Rest_Distance_Greater_Than_Or_Equal_Threshold/End_Point_Number_Calculate ==
  Bus Element In3 : Inport  PortName=input_bus  Element=global_trajectory_cumulative_length
  Bus Element In1 : Inport  PortName=input_bus  Element=global_trajectory_cumulative_length
  Bus Element In2 : Inport  PortName=input_bus  Element=closest_segment_start_point_index_current
  Bus Element In4 : Inport  PortName=input_bus  Element=closest_segment_start_point_index_current
  Bus Element In5 : Inport  PortName=input_bus  Element=global_trajectory_point_number
  IC : Inport  Port=2
  AND : Logic  IconShape=distinctive  AllPortsSameDT=off  OutDataTypeStr=boolean
  Constant : Constant  OutDataTypeStr=int32  SampleTime=-1
  Constant13 : Constant  Value=MAX_TRAJECTORY_LENGTH  OutDataTypeStr=double  SampleTime=-1
  GreaterThan : RelationalOperator  Operator=>  OutDataTypeStr=boolean  RndMeth=Simplest
  LessThanOrEqual : RelationalOperator  Operator=<=  OutDataTypeStr=boolean  RndMeth=Simplest
  Plus : Sum
  Plus1 : Sum
  Selector : Selector  IndexOptions=Index vector (port)  Indices=[1 3]  OutputSizes=1
  Selector1 : Selector  IndexOptions=Index vector (port)  Indices=[1 3]  OutputSizes=1
  Subtract1 : Sum  Inputs=+-
  While Iterator : WhileIterator  MaxIters=MAX_GLOBAL_TRAJECTORY_WAY_POINT_NUMBER  ResetStates=reset  ShowIterationPort=on
  way_point_number : Outport  Description=满足导出轨迹累计弧长条件的从最近点往后的点数。  OutDataTypeStr=int32
  wires:
  IC/1 -> While Iterator/2
  Bus Element In3/1 -> Selector/1
  While Iterator/1 -> Subtract1/1, Plus1/2  "temp_index"
  Constant13/1 -> Plus/1
  Plus/1 -> GreaterThan/1
  Selector/1 -> GreaterThan/2
  Constant/1 -> Subtract1/2
  Subtract1/1 -> way_point_number/1  "temp_index"
  Bus Element In1/1 -> Selector1/1
  Bus Element In2/1 -> Selector1/2
  Selector1/1 -> Plus/2
  Bus Element In4/1 -> Plus1/1
  Plus1/1 -> Selector/2, LessThanOrEqual/1
  GreaterThan/1 -> AND/1
  Bus Element In5/1 -> LessThanOrEqual/2
  LessThanOrEqual/1 -> AND/2
  AND/1 -> While Iterator/1

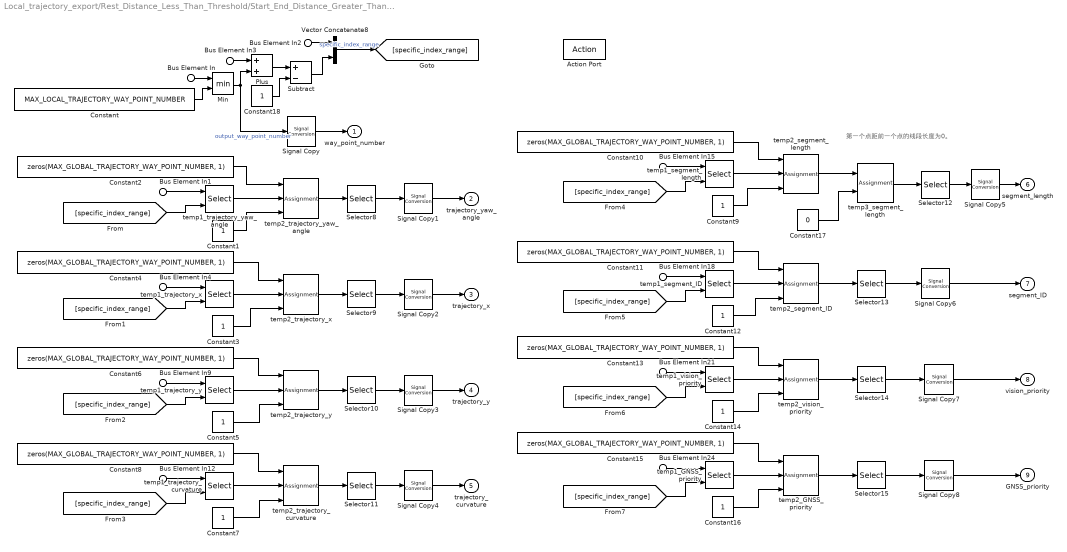
== system Local_trajectory_export/Rest_Distance_Less_Than_Threshold/Start_End_Distance_Greater_Than_Threshold ==
  note: 第一个点距前一个点的线段长度为0。
  Bus Element In : Inport  PortName=input_bus  Element=rest_point_number
  Bus Element In1 : Inport  PortName=input_bus  Element=global_trajectory_yaw_angle
  Bus Element In2 : Inport  PortName=input_bus  Element=closest_segment_start_point_index_current
  Bus Element In3 : Inport  PortName=input_bus  Element=closest_segment_start_point_index_current
  Bus Element In4 : Inport  PortName=input_bus  Element=global_trajectory_x
  Bus Element In9 : Inport  PortName=input_bus  Element=global_trajectory_y
  Bus Element In12 : Inport  PortName=input_bus  Element=global_trajectory_curvature
  Bus Element In15 : Inport  PortName=input_bus  Element=global_trajectory_segment_length
  Bus Element In18 : Inport  PortName=input_bus  Element=global_trajectory_segment_ID
  Bus Element In21 : Inport  PortName=input_bus  Element=global_trajectory_vision_priority
  Bus Element In24 : Inport  PortName=input_bus  Element=global_trajectory_GNSS_priority
  Action Port : ActionPort  PropagateVarSize=During execution  ActionPortLabel=if(u1 < u2)
  Constant : Constant  Value=MAX_LOCAL_TRAJECTORY_WAY_POINT_NUMBER  VectorParams1D=off  OutDataTypeStr=int32  SampleTime=-1
  Constant{1,3,5,7,9,12,14,16,18} (9 alike) : Constant  OutDataTypeStr=int32  SampleTime=-1
  Constant{2,4,6,8,10} (5 alike) : Constant  Value=zeros(MAX_GLOBAL_TRAJECTORY_WAY_POINT_NUMBER, 1)  OutDataTypeStr=double  SampleTime=-1
  Constant11 : Constant  Value=zeros(MAX_GLOBAL_TRAJECTORY_WAY_POINT_NUMBER, 1)  OutDataTypeStr=int8  SampleTime=-1
  Constant13 : Constant  Value=zeros(MAX_GLOBAL_TRAJECTORY_WAY_POINT_NUMBER, 1)  OutDataTypeStr=int8  SampleTime=-1
  Constant15 : Constant  Value=zeros(MAX_GLOBAL_TRAJECTORY_WAY_POINT_NUMBER, 1)  OutDataTypeStr=int8  SampleTime=-1
  Constant17 : Constant  Value=0  OutDataTypeStr=double  SampleTime=-1
  Min : MinMax  Inputs=2  OutDataTypeStr=int32
  Plus : Sum
  Selector{8..15} (8 alike) : Selector  IndexOptions=Starting index (dialog)  Indices=1  OutputSizes=MAX_LOCAL_TRAJECTORY_WAY_POINT_NUMBER
  Signal Copy{,1..8} (9 alike) : SignalConversion  OverrideOpt=off
  Subtract : Sum  Inputs=+-
  Vector Concatenate8 : Concatenate
  temp1_GNSS_priority : Selector  IndexOptions=Starting and ending indices (port)  Indices=[1 3]  OutputSizes=MAX_LOCAL_TRAJECTORY_WAY_POINT_NUMBER
  temp1_segment_ID : Selector  IndexOptions=Starting and ending indices (port)  Indices=[1 3]  OutputSizes=MAX_LOCAL_TRAJECTORY_WAY_POINT_NUMBER
  temp1_segment_length : Selector  IndexOptions=Starting and ending indices (port)  Indices=[1 3]  OutputSizes=MAX_LOCAL_TRAJECTORY_WAY_POINT_NUMBER
  temp1_trajectory_curvature : Selector  IndexOptions=Starting and ending indices (port)  Indices=[1 3]  OutputSizes=MAX_LOCAL_TRAJECTORY_WAY_POINT_NUMBER
  temp1_trajectory_x : Selector  IndexOptions=Starting and ending indices (port)  Indices=[1 3]  OutputSizes=MAX_LOCAL_TRAJECTORY_WAY_POINT_NUMBER
  temp1_trajectory_y : Selector  IndexOptions=Starting and ending indices (port)  Indices=[1 3]  OutputSizes=MAX_LOCAL_TRAJECTORY_WAY_POINT_NUMBER
  temp1_trajectory_yaw_angle : Selector  IndexOptions=Starting and ending indices (port)  Indices=[1 3]  OutputSizes=MAX_LOCAL_TRAJECTORY_WAY_POINT_NUMBER
  temp1_vision_priority : Selector  IndexOptions=Starting and ending indices (port)  Indices=[1 3]  OutputSizes=MAX_LOCAL_TRAJECTORY_WAY_POINT_NUMBER
  temp2_GNSS_priority : Assignment  DiagnosticForDimensions=Warning  IndexOptions=Starting index (port)  Indices=1  OutputSizes=MAX_LOCAL_TRAJECTORY_WAY_POINT_NUMBER
  temp2_segment_ID : Assignment  DiagnosticForDimensions=Warning  IndexOptions=Starting index (port)  Indices=1  OutputSizes=MAX_LOCAL_TRAJECTORY_WAY_POINT_NUMBER
  temp2_segment_length : Assignment  DiagnosticForDimensions=Warning  IndexOptions=Starting index (port)  Indices=1  OutputSizes=MAX_LOCAL_TRAJECTORY_WAY_POINT_NUMBER
  temp2_trajectory_curvature : Assignment  DiagnosticForDimensions=Warning  IndexOptions=Starting index (port)  Indices=1  OutputSizes=MAX_LOCAL_TRAJECTORY_WAY_POINT_NUMBER
  temp2_trajectory_x : Assignment  DiagnosticForDimensions=Warning  IndexOptions=Starting index (port)  Indices=1  OutputSizes=MAX_LOCAL_TRAJECTORY_WAY_POINT_NUMBER
  temp2_trajectory_y : Assignment  DiagnosticForDimensions=Warning  IndexOptions=Starting index (port)  Indices=1  OutputSizes=MAX_LOCAL_TRAJECTORY_WAY_POINT_NUMBER
  temp2_trajectory_yaw_angle : Assignment  DiagnosticForDimensions=Warning  IndexOptions=Starting index (port)  Indices=1  OutputSizes=MAX_LOCAL_TRAJECTORY_WAY_POINT_NUMBER
  temp2_vision_priority : Assignment  DiagnosticForDimensions=Warning  IndexOptions=Starting index (port)  Indices=1  OutputSizes=MAX_LOCAL_TRAJECTORY_WAY_POINT_NUMBER
  temp3_segment_length : Assignment  Description=第一个点距前一个点的线段长度为0。  OutputInitialize=Specify size for each dimension in table  DiagnosticForDimensions=Warning  IndexOptions=Index vector (dialog)  Indices=1  OutputSizes=MAX_LOCAL_TRAJECTORY_WAY_POINT_NUMBER
  way_point_number : Outport  Description=导出的局部轨迹有效路点个数，自然数，无量纲。  OutDataTypeStr=int32  PortDimensions=1
  trajectory_yaw_angle : Outport  Description=导出的局部轨迹横摆角数组，有效数据数量为way_point_number，其余补零，实数，deg。  Port=2  OutDataTypeStr=double  PortDimensions=MAX_LOCAL_TRAJECTORY_WAY_POINT_NUMBER
  trajectory_x : Outport  Description=导出的局部轨迹x坐标数组，有效数据数量为way_point_number，其余补零，实数，m。  Port=3  OutDataTypeStr=double  PortDimensions=MAX_LOCAL_TRAJECTORY_WAY_POINT_NUMBER
  trajectory_y : Outport  Description=导出的局部轨迹y坐标数组，有效数据数量为way_point_number，其余补零，实数，m。  Port=4  OutDataTypeStr=double  PortDimensions=MAX_LOCAL_TRAJECTORY_WAY_POINT_NUMBER
  trajectory_curvature : Outport  Description=导出的局部轨迹曲率数组，有效数据数量为way_point_number，其余补零，实数，1/m。  Port=5  OutDataTypeStr=double  PortDimensions=MAX_LOCAL_TRAJECTORY_WAY_POINT_NUMBER
  segment_length : Outport  Description=导出的局部轨迹路点到前一个点的线段长度数组，有效数据数量为way_point_number，其余补零，正实数，m。  Port=6  OutDataTypeStr=double  PortDimensions=MAX_LOCAL_TRAJECTORY_WAY_POINT_NUMBER
  segment_ID : Outport  Description=导出的局部轨迹区间代号数组，有效数据数量为way_point_number，其余补零，正整数，无量纲。  Port=7  OutDataTypeStr=int8  PortDimensions=MAX_LOCAL_TRAJECTORY_WAY_POINT_NUMBER
  vision_priority : Outport  Description=导出的局部轨迹视觉循迹优先级数组，有效数据数量为way_point_number，其余补零，自然数，无量纲。  Port=8  OutDataTypeStr=int8  PortDimensions=MAX_LOCAL_TRAJECTORY_WAY_POINT_NUMBER
  GNSS_priority : Outport  Description=导出的局部轨迹GNSS循迹优先级数组，有效数据数量为way_point_number，其余补零，自然数，无量纲。  Port=9  OutDataTypeStr=int8  PortDimensions=MAX_LOCAL_TRAJECTORY_WAY_POINT_NUMBER
  wires:
  Bus Element In/1 -> Min/1
  Constant/1 -> Min/2
  Min/1 -> Plus/2, Signal Copy/1  "output_way_point_number"
  Bus Element In1/1 -> temp1_trajectory_yaw_angle/1
  Bus Element In4/1 -> temp1_trajectory_x/1
  Bus Element In9/1 -> temp1_trajectory_y/1
  temp1_trajectory_y/1 -> temp2_trajectory_y/2
  Constant5/1 -> temp2_trajectory_y/3
  Constant7/1 -> temp2_trajectory_curvature/3
  temp1_trajectory_curvature/1 -> temp2_trajectory_curvature/2
  Bus Element In12/1 -> temp1_trajectory_curvature/1
  Bus Element In15/1 -> temp1_segment_length/1
  Constant9/1 -> temp2_segment_length/3
  Constant12/1 -> temp2_segment_ID/3
  Bus Element In18/1 -> temp1_segment_ID/1
  Constant14/1 -> temp2_vision_priority/3
  Constant16/1 -> temp2_GNSS_priority/3
  Bus Element In24/1 -> temp1_GNSS_priority/1
  Selector15/1 -> Signal Copy8/1
  temp2_trajectory_yaw_angle/1 -> Selector8/1
  Selector9/1 -> Signal Copy2/1
  Selector14/1 -> Signal Copy7/1
  Selector13/1 -> Signal Copy6/1
  Bus Element In2/1 -> Vector Concatenate8/1
  Subtract/1 -> Vector Concatenate8/2
  Vector Concatenate8/1 -> [specific_index_range]  "specific_index_range"
  [specific_index_range] -> temp1_trajectory_yaw_angle/2
  temp1_trajectory_yaw_angle/1 -> temp2_trajectory_yaw_angle/2
  Constant1/1 -> temp2_trajectory_yaw_angle/3
  Constant2/1 -> temp2_trajectory_yaw_angle/1
  [specific_index_range] -> temp1_trajectory_x/2
  temp1_trajectory_x/1 -> temp2_trajectory_x/2
  Constant3/1 -> temp2_trajectory_x/3
  temp2_trajectory_x/1 -> Selector9/1
  Constant4/1 -> temp2_trajectory_x/1
  [specific_index_range] -> temp1_trajectory_y/2
  Constant6/1 -> temp2_trajectory_y/1
  Selector10/1 -> Signal Copy3/1
  temp2_trajectory_y/1 -> Selector10/1
  [specific_index_range] -> temp1_trajectory_curvature/2
  Constant8/1 -> temp2_trajectory_curvature/1
  temp2_trajectory_curvature/1 -> Selector11/1
  Selector11/1 -> Signal Copy4/1
  [specific_index_range] -> temp1_segment_length/2
  temp1_segment_length/1 -> temp2_segment_length/2
  Constant10/1 -> temp2_segment_length/1
  temp2_segment_length/1 -> temp3_segment_length/1
  Constant17/1 -> temp3_segment_length/2
  temp3_segment_length/1 -> Selector12/1
  Selector12/1 -> Signal Copy5/1
  [specific_index_range] -> temp1_segment_ID/2
  temp1_segment_ID/1 -> temp2_segment_ID/2
  Constant11/1 -> temp2_segment_ID/1
  temp2_segment_ID/1 -> Selector13/1
  Bus Element In21/1 -> temp1_vision_priority/1
  [specific_index_range] -> temp1_vision_priority/2
  temp1_vision_priority/1 -> temp2_vision_priority/2
  Constant13/1 -> temp2_vision_priority/1
  temp2_vision_priority/1 -> Selector14/1
  [specific_index_range] -> temp1_GNSS_priority/2
  temp1_GNSS_priority/1 -> temp2_GNSS_priority/2
  Constant15/1 -> temp2_GNSS_priority/1
  temp2_GNSS_priority/1 -> Selector15/1
  Bus Element In3/1 -> Plus/1
  Plus/1 -> Subtract/1
  Constant18/1 -> Subtract/2
  Selector8/1 -> Signal Copy1/1
  Signal Copy/1 -> way_point_number/1
  Signal Copy1/1 -> trajectory_yaw_angle/1
  Signal Copy2/1 -> trajectory_x/1
  Signal Copy3/1 -> trajectory_y/1
  Signal Copy4/1 -> trajectory_curvature/1
  Signal Copy5/1 -> segment_length/1
  Signal Copy6/1 -> segment_ID/1
  Signal Copy7/1 -> vision_priority/1
  Signal Copy8/1 -> GNSS_priority/1
